simulink model "speed_control"  (R2024a)
settings: Solver=VariableStepAuto  StartTime=0.0  StopTime=90  MaxStep=0.01  RelTol=1e-3
values from neighbouring files (symbols this model uses):
  F_max = 15    [init.m]
  F_min = -15    [init.m]
  K = ki*tau - kd/tau    (= -49.7)    [init.m]
  k = 0.5    [init.m]
  kbc = 1/(kp+kd/tau)    (= 0.0142857142857)    [init.m]
  kd = 5    [init.m]
  ki = 3    [init.m]
  kp = 20    [init.m]
  m = 10    [init.m]
  T = 0.1    [init.m]
  tau = 0.1    [init.m]
undefined symbols (not defined in the file or in its folder): DiscIntNeverNeededParam
settings Model: Creator=berto  LastModifiedBy=berto

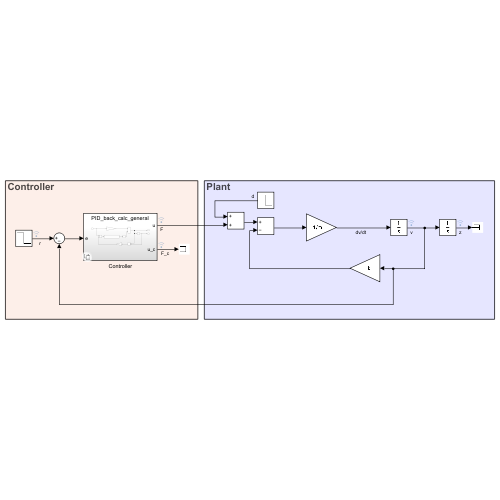
[thumbnail: Simulink's stored preview of the top-level diagram]
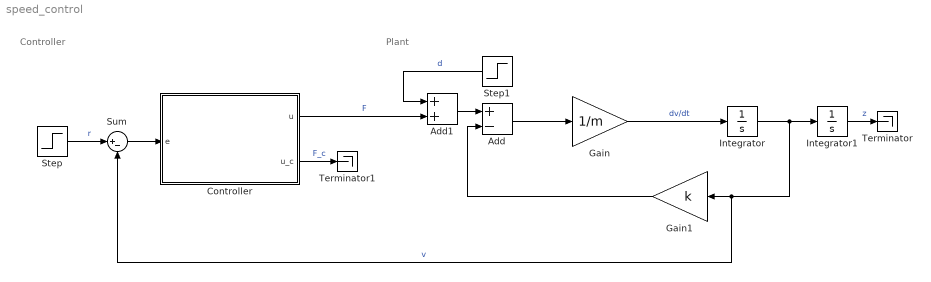
== system speed_control ==
  note: Controller
  note: Plant
  Add : Sum  Inputs=+-
  Add1 : Sum
  Controller : Subsystem  Variant=on
  Gain : Gain  Gain=1/m
  Gain1 : Gain  Gain=k
  Integrator : Integrator
  Integrator1 : Integrator
  Step : Step  Time=30  Before=20  After=10  SampleTime=0
  Step1 : Step  Time=60  After=-8  SampleTime=0
  Sum : Sum  Inputs=|+-
  Terminator : Terminator
  Terminator1 : Terminator
  wires:
  Controller/1(u) -> Add1/2  "F"
  Step/1 -> Sum/1  "r"
  Sum/1 -> Controller/1(e)
  Add/1 -> Gain/1
  Gain/1 -> Integrator/1  "dv/dt"
  Integrator/1 -> Sum/2, Gain1/1, Integrator1/1  "v"
  Gain1/1 -> Add/2
  Step1/1 -> Add1/1  "d"
  Add1/1 -> Add/1
  Integrator1/1 -> Terminator/1  "z"
  Controller/2(u_c) -> Terminator1/1  "F_c"

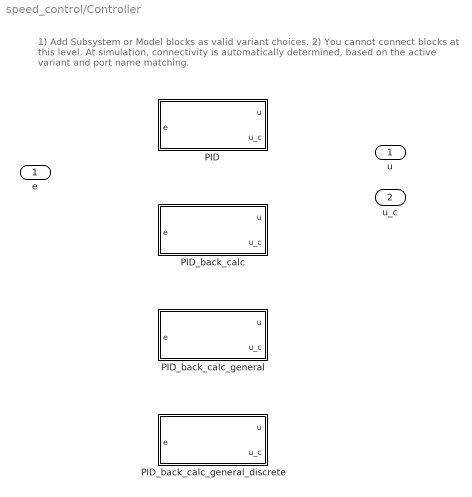
== system speed_control/Controller ==
  note: 1) Add Subsystem or Model blocks as valid variant choices.
      | 2) You cannot connect blocks at this level. At simulation, connectivity is automatically
      | determined, based on the active variant and port name matching.
  e : Inport
  PID : Subsystem  VariantControl=ctrl_type == 0
  PID_back_calc : Subsystem  VariantControl=ctrl_type == 1
  PID_back_calc_general : Subsystem  VariantControl=ctrl_type == 3
  PID_back_calc_general_discrete : Subsystem  VariantControl=ctrl_type == 4
  u : Outport
  u_c : Outport  Port=2

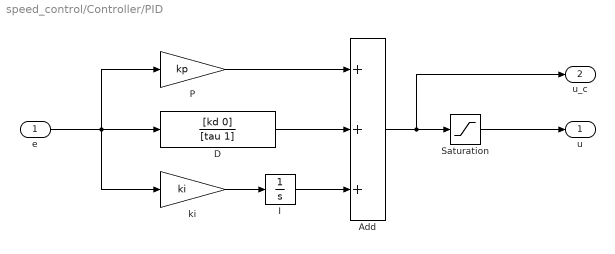
== system speed_control/Controller/PID ==
  e : Inport
  Add : Sum  Inputs=+++
  D : TransferFcn  Numerator=[kd 0]  Denominator=[tau 1]
  I : Integrator
  P : Gain  Gain=kp
  Saturation : Saturate  UpperLimit=F_max  LowerLimit=F_min
  ki : Gain  Gain=ki
  u : Outport
  u_c : Outport  Port=2
  wires:
  ki/1 -> I/1
  Add/1 -> u_c/1, Saturation/1
  D/1 -> Add/2
  I/1 -> Add/3
  P/1 -> Add/1
  e/1 -> ki/1, P/1, D/1
  Saturation/1 -> u/1

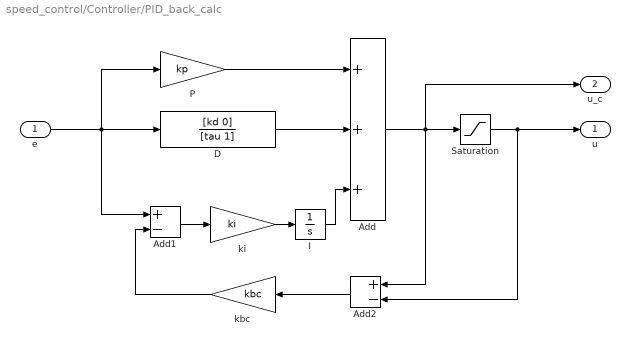
== system speed_control/Controller/PID_back_calc ==
  e : Inport
  Add : Sum  Inputs=+++
  Add1 : Sum  Inputs=+-
  Add2 : Sum  Inputs=+-
  D : TransferFcn  Numerator=[kd 0]  Denominator=[tau 1]
  I : Integrator
  P : Gain  Gain=kp
  Saturation : Saturate  UpperLimit=F_max  LowerLimit=F_min
  kbc : Gain  Gain=kbc
  ki : Gain  Gain=ki
  u : Outport
  u_c : Outport  Port=2
  wires:
  Add/1 -> u_c/1, Add2/1, Saturation/1
  e/1 -> Add1/1, P/1, D/1
  D/1 -> Add/2
  P/1 -> Add/1
  Saturation/1 -> Add2/2, u/1
  kbc/1 -> Add1/2
  Add2/1 -> kbc/1
  I/1 -> Add/3
  ki/1 -> I/1
  Add1/1 -> ki/1

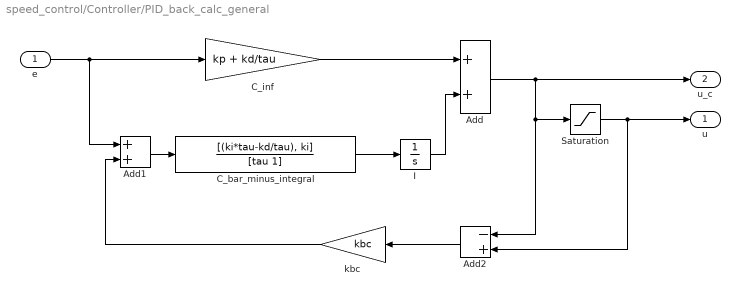
== system speed_control/Controller/PID_back_calc_general ==
  e : Inport
  Add : Sum
  Add1 : Sum
  Add2 : Sum  Inputs=-+
  C_bar_minus_integral : TransferFcn  Numerator=[(ki*tau-kd/tau), ki]  Denominator=[tau 1]
  C_inf : Gain  Gain=kp + kd/tau
  I : Integrator
  Saturation : Saturate  UpperLimit=F_max  LowerLimit=F_min
  kbc : Gain  Gain=kbc
  u : Outport
  u_c : Outport  Port=2
  wires:
  Add/1 -> u_c/1, Add2/1, Saturation/1
  e/1 -> Add1/1, C_inf/1
  Saturation/1 -> Add2/2, u/1
  Add2/1 -> kbc/1
  kbc/1 -> Add1/2
  C_inf/1 -> Add/1
  I/1 -> Add/2
  Add1/1 -> C_bar_minus_integral/1
  C_bar_minus_integral/1 -> I/1

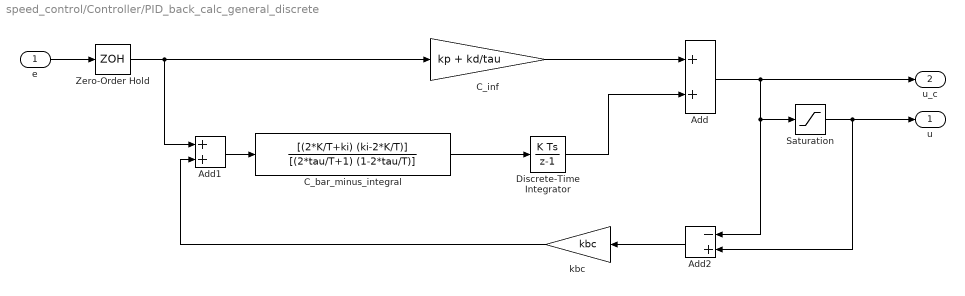
== system speed_control/Controller/PID_back_calc_general_discrete ==
  e : Inport
  Add : Sum
  Add1 : Sum
  Add2 : Sum  Inputs=-+
  C_bar_minus_integral : DiscreteTransferFcn  Numerator=[(2*K/T+ki) (ki-2*K/T)]  Denominator=[(2*tau/T+1) (1-2*tau/T)]
  C_inf : Gain  Gain=kp + kd/tau
  Discrete-Time Integrator : DiscreteIntegrator  SampleTime=T  ICPrevOutput=DiscIntNeverNeededParam  ICPrevScaledInput=DiscIntNeverNeededParam
  Saturation : Saturate  UpperLimit=F_max  LowerLimit=F_min
  Zero-Order Hold : ZeroOrderHold  SampleTime=T
  kbc : Gain  Gain=kbc
  u : Outport
  u_c : Outport  Port=2
  wires:
  C_bar_minus_integral/1 -> Discrete-Time Integrator/1
  Add1/1 -> C_bar_minus_integral/1
  Discrete-Time Integrator/1 -> Add/2
  C_inf/1 -> Add/1
  kbc/1 -> Add1/2
  Add2/1 -> kbc/1
  Saturation/1 -> u/1, Add2/2
  e/1 -> Zero-Order Hold/1
  Add/1 -> Saturation/1, Add2/1, u_c/1
  Zero-Order Hold/1 -> C_inf/1, Add1/1
